simulink model "servo"  (R2014a)
settings: Solver=VariableStepAuto  StartTime=0.0  StopTime=30  RelTol=1e-3
values from neighbouring files (symbols this model uses):
  A = [0 1; -a0 -a1]    [MISO_main.m]    (also in boost_ss.m = [0 -(1-d)/l; (1-d)/c -1/r*c])
  B = [0 ; 1]    [MISO_main.m]    (also in boost_ss.m = [1/l vc_eqm/l; 0 -il_eqm/c])
  C = [b0 b1]    [MISO_main.m]    (also in boost_ss.m = [0 1])
  D = 0    [MISO_main.m]    (also in boost_ss.m = [0])
  Gc = -1/(C*(Ac)^-1*B)    [tracking_MISO.m]
undefined symbols (not defined in the file or in its folder): Ksrv, Kt, x0
settings Model: Creator=Bara  LastModifiedBy=Administrator
settings DataIOCC: LimitDataPoints=off  SaveFormat=Dataset
settings OptimizationCC: SimCompilerOptimization=off
settings DebuggingCC: MergeDetectMultiDrivingBlocksExec=error  SolverPrmCheckMsg=none  FrameProcessingCompatibilityMsg=error
settings HardwareCC: ProdBitPerPointer=64  ProdLargestAtomicFloat=Float  ProdIntDivRoundTo=Zero  ProdEndianess=LittleEndian  ProdWordSize=64  ProdHWDeviceType=Intel->x86-64 (Windows64)
settings ModelReferenceCC: PropagateSignalLabelsOutOfModel=on
settings RTWCC: RTWCompilerOptimization=off
settings ConfigComp: CovMetricSettings=dw  CovHtmlReporting=on  CovSaveCumulativeToWorkspaceVar=on  CovSaveSingleToWorkspaceVar=on  CovExternalEMLEnable=off

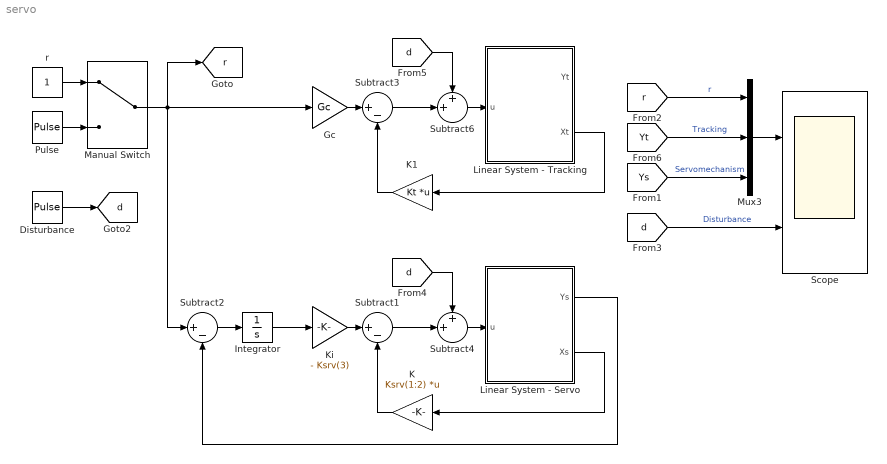
== system servo ==
  Disturbance : DiscretePulseGenerator  PulseType=Time based  Amplitude=0.5  Period=50  PulseWidth=50
  Gc : Gain  Gain=Gc
  Integrator : Integrator  InitialCondition=C*x0
  K : Gain  Gain=Ksrv(1:2)  Multiplication=Matrix(K*u) (u vector)
  K1 : Gain  Gain=Kt  Multiplication=Matrix(K*u) (u vector)
  Ki : Gain  Gain=- Ksrv(3)
  Linear System - Servo : Subsystem
  Linear System - Tracking : Subsystem
  Manual Switch : ManualSwitch
  Mux3 : Mux  Inputs=3
  Pulse : DiscretePulseGenerator  PulseType=Time based  Period=20  PulseWidth=50
  Scope : Scope  NumInputPorts=2
      settings: TickLabels=on  ShowLegends=on  YMin=0~-0.7  YMax=105~0.7
  Subtract1 : Sum  Inputs=|+-
  Subtract2 : Sum  Inputs=|+-
  Subtract3 : Sum  Inputs=|+-
  Subtract4 : Sum  Inputs=++|
  Subtract6 : Sum  Inputs=++|
  r : Constant
  tag scope: d=global, r=global
  wires:
  Mux3/1 -> Scope/1
  [Ys] -> Mux3/3  "Servomechanism"
  [r] -> Mux3/1  "r"
  r/1 -> Manual Switch/1
  Pulse/1 -> Manual Switch/2
  Linear System - Servo/2(Xs) -> K/1
  K/1 -> Subtract1/2
  Subtract1/1 -> Subtract4/2
  Ki/1 -> Subtract1/1
  Integrator/1 -> Ki/1
  Subtract2/1 -> Integrator/1
  Linear System - Servo/1(Ys) -> Subtract2/2
  Subtract4/1 -> Linear System - Servo/1(u)
  [d] -> Scope/2  "Disturbance"
  Disturbance/1 -> [d]
  [d] -> Subtract4/1
  Linear System - Tracking/2(Xt) -> K1/1
  K1/1 -> Subtract3/2
  Subtract3/1 -> Subtract6/2
  Gc/1 -> Subtract3/1
  Manual Switch/1 -> Gc/1, [r], Subtract2/1
  Subtract6/1 -> Linear System - Tracking/1(u)
  [d] -> Subtract6/1
  [Yt] -> Mux3/2  "Tracking"

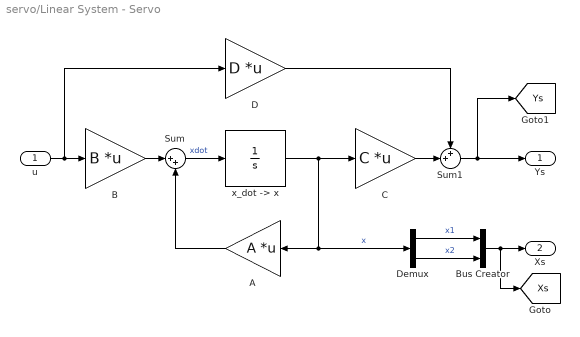
== system servo/Linear System - Servo ==
  u : Inport
  A : Gain  Gain=A  Multiplication=Matrix(K*u) (u vector)
  B : Gain  Gain=B  Multiplication=Matrix(K*u) (u vector)
  Bus Creator : BusCreator  Inputs=2
  C : Gain  Gain=C  Multiplication=Matrix(K*u) (u vector)
  D : Gain  Gain=D  Multiplication=Matrix(K*u) (u vector)
  Demux : Demux  Outputs=2
  Sum : Sum  Inputs=|++
  Sum1 : Sum  Inputs=++|
  "x_dot -> x" : Integrator  InitialCondition=x0
  Ys : Outport
  Xs : Outport  Port=2
  tag scope: Xs=global, Ys=global
  wires:
  Bus Creator/1 -> [Xs], Xs/1
  Demux/2 -> Bus Creator/2  "x2"
  Demux/1 -> Bus Creator/1  "x1"
  Sum1/1 -> Ys/1, [Ys]
  D/1 -> Sum1/1
  C/1 -> Sum1/2
  u/1 -> B/1, D/1
  B/1 -> Sum/1
  A/1 -> Sum/2
  "x_dot -> x"/1 -> C/1, A/1, Demux/1  "x"
  Sum/1 -> "x_dot -> x"/1  "xdot"

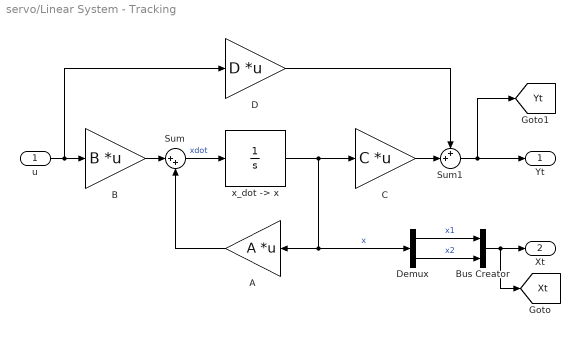
== system servo/Linear System - Tracking ==
  u : Inport
  A : Gain  Gain=A  Multiplication=Matrix(K*u) (u vector)
  B : Gain  Gain=B  Multiplication=Matrix(K*u) (u vector)
  Bus Creator : BusCreator  Inputs=2
  C : Gain  Gain=C  Multiplication=Matrix(K*u) (u vector)
  D : Gain  Gain=D  Multiplication=Matrix(K*u) (u vector)
  Demux : Demux  Outputs=2
  Sum : Sum  Inputs=|++
  Sum1 : Sum  Inputs=++|
  "x_dot -> x" : Integrator  InitialCondition=x0
  Yt : Outport
  Xt : Outport  Port=2
  tag scope: Xt=global, Yt=global
  wires:
  Sum/1 -> "x_dot -> x"/1  "xdot"
  "x_dot -> x"/1 -> Demux/1, A/1, C/1  "x"
  A/1 -> Sum/2
  B/1 -> Sum/1
  u/1 -> D/1, B/1
  C/1 -> Sum1/2
  D/1 -> Sum1/1
  Sum1/1 -> [Yt], Yt/1
  Demux/1 -> Bus Creator/1  "x1"
  Bus Creator/1 -> Xt/1, [Xt]
  Demux/2 -> Bus Creator/2  "x2"
